simulink model "cruise_control_model"  (R2024a)
settings: Solver=ode45  StartTime=0.0  StopTime=T  MaxStep=0.1  RelTol=1e-3  EnableMultiTasking=on
PreLoadFcn:
  | m = 1000;
  | alpha = [40, 25, 16, 12, 10];
  | Tm = 190;
  | wm = 420;
  | beta = 0.4;
  | Cr = 0.01;
  | rho = 1.3;
  | Cd = 0.32;
  | A = 2.4;
  | g = 9.8;
  | theta = 0;
  | gear = 3;
undefined symbols (not defined in the file or in its folder): ki, kp
libraries: simulink x1
settings Model: Creator=Cole Lepine  LastModifiedBy=marmr
settings SolverCC: AlgebraicLoopSolver=TrustRegion
settings DataIOCC: LimitDataPoints=on  SaveFormat=Array  SignalLoggingSaveFormat=ModelDataLogs  ReturnWorkspaceOutputs=off
settings OptimizationCC: ReuseModelBlockBuffer=off  ExpressionDepthLimit=2147483647  InitFltsAndDblsToZero=on  LifeSpan=inf
settings DebuggingCC: UnderspecifiedInitializationDetection=Classic  MergeDetectMultiDrivingBlocksExec=none  SolverPrmCheckMsg=warning  FcnCallInpInsideContextMsg=warning  UnconnectedInputMsg=warning  UnconnectedOutputMsg=warning  UnconnectedLineMsg=warning  StateNameClashWarn=warning  SFUnexpectedBacktrackingDiag=warning  SFNoUnconditionalDefaultTransitionDiag=warning  SFExecutionAtInitializationDiag=none  ArithmeticOperatorsInVariantConditions=warning
settings HardwareCC: ProdBitPerPointer=32  ProdBitPerSizeT=32  ProdBitPerPtrDiffT=32  ProdLargestAtomicFloat=None  ProdIntDivRoundTo=Undefined  ProdEndianess=Unspecified  ProdWordSize=32  ProdHWDeviceType=32-bit Generic
settings ModelReferenceCC: PropagateSignalLabelsOutOfModel=off
settings RTWCC: GPUComputeCapability=3.5
settings CodeAppCC: StateflowObjectComments=on
settings GRTTargetCC: TargetLangStandard=C89/C90 (ANSI)  CombineOutputUpdateFcns=off  GRTInterface=on
settings ConfigComp: CovMetricSettings=dw  CovSaveCumulativeToWorkspaceVar=on  CovSaveSingleToWorkspaceVar=on

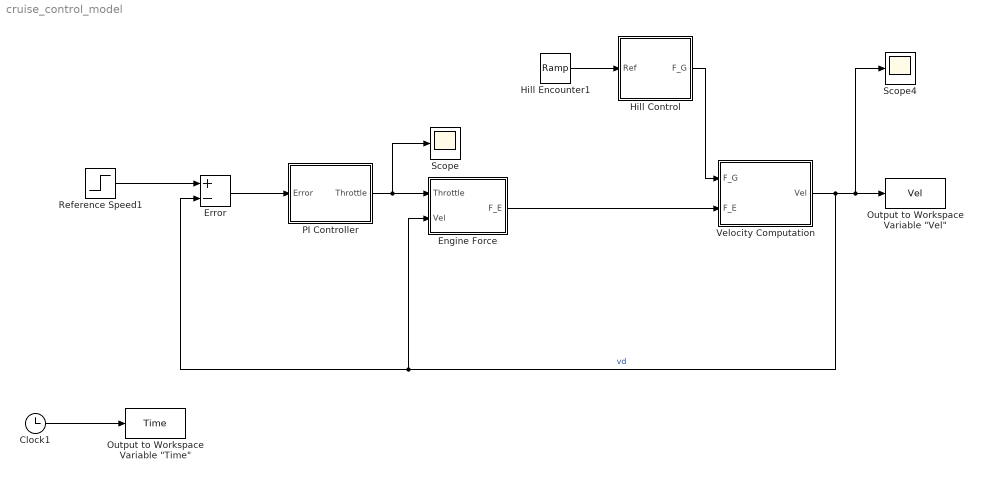
== system cruise_control_model ==
  Clock1 : Clock
  Engine Force : Subsystem
  Error : Sum  Inputs=+-
  Hill Control : Subsystem
  Hill Encounter1 : simulink/Sources/Ramp  slope=1  start=120  InitialOutput=0
  "Output to Workspace Variable \"Time\"" : ToWorkspace  VariableName=Time  SampleTime=-1
      settings: Decimation=2
  "Output to Workspace Variable \"Vel\"" : ToWorkspace  VariableName=Vel  SampleTime=-1
      settings: Decimation=2
  PI Controller : Subsystem
  Reference Speed1 : Step  Time=20  Before=20  After=30  SampleTime=0
  Scope : Scope
  Scope4 : Scope
  Velocity Computation : Subsystem
  wires:
  Error/1 -> PI Controller/1(Error)
  Engine Force/1(F_E) -> Velocity Computation/2(F_E)
  Hill Control/1(F_G) -> Velocity Computation/1(F_G)
  Clock1/1 -> "Output to Workspace Variable \"Time\""/1
  Reference Speed1/1 -> Error/1
  PI Controller/1(Throttle) -> Scope/1, Engine Force/1(Throttle)
  Hill Encounter1/1 -> Hill Control/1(Ref)
  Velocity Computation/1(Vel) -> Error/2, Engine Force/2(Vel), Scope4/1, "Output to Workspace Variable \"Vel\""/1  "vd"

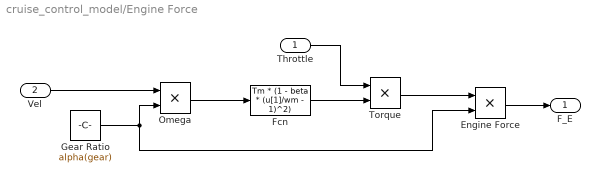
== system cruise_control_model/Engine Force ==
  Throttle : Inport
  Vel : Inport  Port=2
  Engine Force : Product  Inputs=**
  Fcn : Fcn  Expr=Tm * (1 - beta * (u[1]/wm - 1)^2)
  Gear Ratio : Constant  Value=alpha(gear)
  Omega : Product  RndMeth=Zero
  Torque : Product  RndMeth=Zero
  F_E : Outport
  wires:
  Engine Force/1 -> F_E/1
  Omega/1 -> Fcn/1
  Gear Ratio/1 -> Omega/2, Engine Force/2
  Torque/1 -> Engine Force/1
  Fcn/1 -> Torque/2
  Vel/1 -> Omega/1
  Throttle/1 -> Torque/1

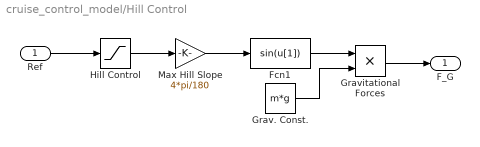
== system cruise_control_model/Hill Control ==
  Ref : Inport
  Fcn1 : Fcn
  Grav. Const. : Constant  Value=m*g
  Gravitational Forces : Product  RndMeth=Zero
  Hill Control : Saturate  UpperLimit=1  LowerLimit=0
  Max Hill Slope : Gain  Gain=4*pi/180
  F_G : Outport
  wires:
  Ref/1 -> Hill Control/1
  Grav. Const./1 -> Gravitational Forces/2
  Hill Control/1 -> Max Hill Slope/1
  Fcn1/1 -> Gravitational Forces/1
  Gravitational Forces/1 -> F_G/1
  Max Hill Slope/1 -> Fcn1/1

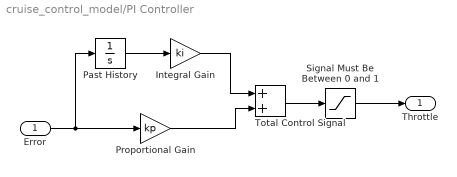
== system cruise_control_model/PI Controller ==
  Error : Inport
  Integral Gain : Gain  Gain=ki
  Past History : Integrator  InitialCondition=1
  Proportional Gain : Gain  Gain=kp
  Signal Must Be Between 0 and 1 : Saturate  UpperLimit=1  LowerLimit=0
  Total Control Signal : Sum
  Throttle : Outport
  wires:
  Signal Must Be Between 0 and 1/1 -> Throttle/1
  Error/1 -> Proportional Gain/1, Past History/1
  Integral Gain/1 -> Total Control Signal/1
  Total Control Signal/1 -> Signal Must Be Between 0 and 1/1
  Past History/1 -> Integral Gain/1
  Proportional Gain/1 -> Total Control Signal/2

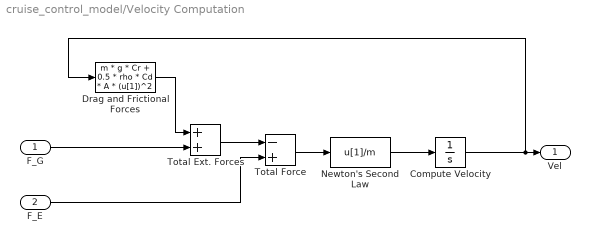
== system cruise_control_model/Velocity Computation ==
  F_G : Inport
  F_E : Inport  Port=2
  Compute Velocity : Integrator  InitialCondition=20
  Drag and Frictional Forces : Fcn  Expr=m * g * Cr + 0.5 * rho * Cd * A * (u[1])^2
  Newton's Second Law : Fcn  Expr=u[1]/m
  Total Ext. Forces : Sum
  Total Force : Sum  Inputs=-+
  Vel : Outport
  wires:
  F_E/1 -> Total Force/2
  Drag and Frictional Forces/1 -> Total Ext. Forces/1
  Newton's Second Law/1 -> Compute Velocity/1
  Total Ext. Forces/1 -> Total Force/1
  Total Force/1 -> Newton's Second Law/1
  Compute Velocity/1 -> Drag and Frictional Forces/1, Vel/1
  F_G/1 -> Total Ext. Forces/2
